simulink model "LQR"  (R2022b)
settings: Solver=VariableStepAuto  StartTime=0.0  StopTime=20  RelTol=1e-3
values from neighbouring files (symbols this model uses):
  B = [0 0 0 0;          1/Jx 0 0 0;          0 0 0 0 ... (first row only)    [config.m]
  g = 9.8    [config.m]
  Jx = 2*Mc*R^2/5 + 2*m*l^2    (= 0.0448)    [config.m]
  Jy = 2*Mc*R^2/5 + 2*m*l^2    (= 0.0448)    [config.m]
  Jz = 2*Mc*R^2/5 + 4*m*l^2    (= 0.0808)    [config.m]
  M = Mc + 4*m    (= 3)    [config.m]
undefined symbols (not defined in the file or in its folder): K_lqr
settings Model: Creator=cxk  LastModifiedBy=cxk

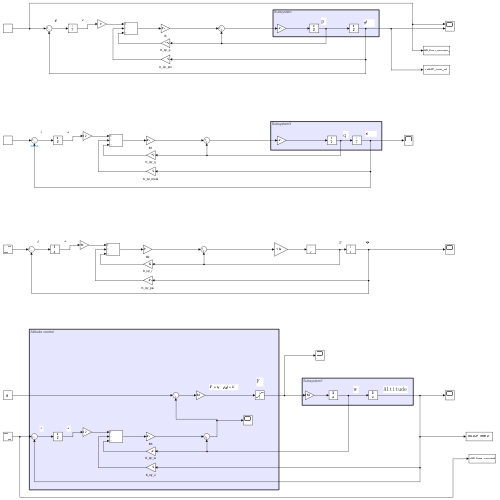
[thumbnail: Simulink's stored preview of the top-level diagram]
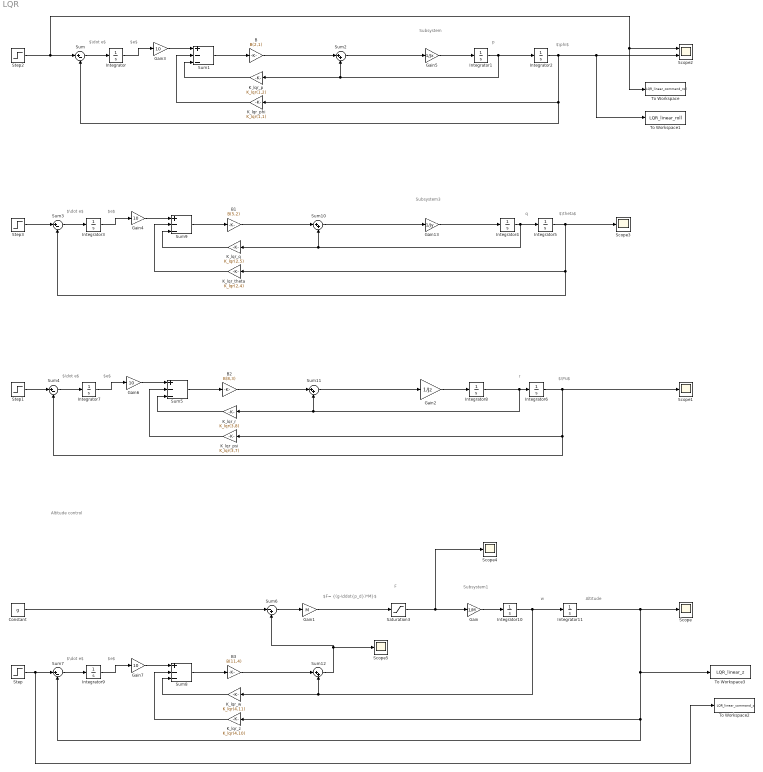
== system LQR ==
  note: Subsystem3
  note: Subsystem
  note: Altitude control
  note: Altitude
  note: $F= {(g-\ddot{p_d})*M}$
  note: Subsystem1
  note: w
  note: F
  note: $\Psi$
  note: r
  note: $\dot e$
  note: $e$
  note: p
  note: $\phi$
  note: $\theta$
  note: q
  note: $\dot e$
  note: $e$
  note: $\dot e$
  note: $e$
  note: $\dot e$
  note: $e$
  B : Gain  Gain=B(2,1)
  B1 : Gain  Gain=B(5,2)
  B2 : Gain  Gain=B(8,3)
  B3 : Gain  Gain=B(11,4)
  Constant : Constant  Value=g
  Gain : Gain  Gain=1/M
  Gain1 : Gain  Gain=M
  Gain13 : Gain  Gain=1/Jy
  Gain2 : Gain  Gain=1/Jz
  Gain{3..4,6..7} (4 alike) : Gain  Gain=10
  Gain5 : Gain  Gain=1/Jx
  Integrator{,1..11} (12 alike) : Integrator
  K_lqr_p : Gain  Gain=K_lqr(1,2)
  K_lqr_phi : Gain  Gain=K_lqr(1,1)
  K_lqr_psi : Gain  Gain=K_lqr(3,7)
  K_lqr_q : Gain  Gain=K_lqr(2,5)
  K_lqr_r : Gain  Gain=K_lqr(3,8)
  K_lqr_theta : Gain  Gain=K_lqr(2,4)
  K_lqr_w : Gain  Gain=K_lqr(4,11)
  K_lqr_z : Gain  Gain=K_lqr(4,10)
  Saturation3 : Saturate  UpperLimit=g*M*10  LowerLimit=-2.97*M*10
  Scope{,1,3..5} (5 alike) : Scope
  Scope2 : Scope  NumInputPorts=2
  Step : Step  After=-3  SampleTime=0
  Step1 : Step  SampleTime=0
  Step2 : Step  After=0.68  SampleTime=0
  Step3 : Step  After=0.68  SampleTime=0
  Sum{,3..4,7} (4 alike) : Sum  Inputs=|+-
  Sum{1,5,8..9} (4 alike) : Sum  Inputs=+--
  Sum{2,10..12} (4 alike) : Sum  Inputs=|++
  Sum6 : Sum  Inputs=|-+
  To Workspace : ToWorkspace  VariableName=LQR_linear_command_roll  SaveFormat=Timeseries  SampleTime=-1
  To Workspace1 : ToWorkspace  VariableName=LQR_linear_roll  SaveFormat=Timeseries  SampleTime=-1
  To Workspace2 : ToWorkspace  VariableName=LQR_linear_command_z  SaveFormat=Timeseries  SampleTime=-1
  To Workspace3 : ToWorkspace  VariableName=LQR_linear_z  SaveFormat=Timeseries  SampleTime=-1
  wires:
  Constant/1 -> Sum6/1
  Saturation3/1 -> Scope4/1, Gain/1
  Gain1/1 -> Saturation3/1
  Gain/1 -> Integrator10/1
  Sum6/1 -> Gain1/1
  Gain2/1 -> Integrator8/1
  Step2/1 -> To Workspace/1, Scope2/1, Sum/1
  Integrator2/1 -> K_lqr_phi/1, Sum/2, To Workspace1/1, Scope2/2
  Sum/1 -> Integrator/1
  Integrator/1 -> Gain3/1
  Gain3/1 -> Sum1/1
  K_lqr_phi/1 -> Sum1/2
  Sum1/1 -> B/1
  Integrator1/1 -> Sum2/2, K_lqr_p/1, Integrator2/1
  Sum2/1 -> Gain5/1
  B/1 -> Sum2/1
  K_lqr_p/1 -> Sum1/3
  Gain13/1 -> Integrator4/1
  Step3/1 -> Sum3/1
  Integrator4/1 -> Integrator5/1, Sum10/2, K_lqr_q/1
  K_lqr_q/1 -> Sum9/3
  Sum10/1 -> Gain13/1
  Sum3/1 -> Integrator3/1
  Integrator3/1 -> Gain4/1
  B1/1 -> Sum10/1
  Sum9/1 -> B1/1
  K_lqr_theta/1 -> Sum9/2
  Integrator5/1 -> K_lqr_theta/1, Sum3/2, Scope3/1
  Gain4/1 -> Sum9/1
  Gain5/1 -> Integrator1/1
  Step1/1 -> Sum4/1
  Integrator8/1 -> Sum11/2, K_lqr_r/1, Integrator6/1
  K_lqr_r/1 -> Sum5/3
  Sum11/1 -> Gain2/1
  Sum4/1 -> Integrator7/1
  Integrator7/1 -> Gain6/1
  B2/1 -> Sum11/1
  Sum5/1 -> B2/1
  K_lqr_psi/1 -> Sum5/2
  Integrator6/1 -> Sum4/2, K_lqr_psi/1, Scope1/1
  Gain6/1 -> Sum5/1
  Integrator10/1 -> Sum12/2, K_lqr_w/1, Integrator11/1
  K_lqr_w/1 -> Sum8/3
  Sum12/1 -> Sum6/2, Scope5/1
  Sum7/1 -> Integrator9/1
  Integrator9/1 -> Gain7/1
  B3/1 -> Sum12/1
  Sum8/1 -> B3/1
  K_lqr_z/1 -> Sum8/2
  Gain7/1 -> Sum8/1
  Integrator11/1 -> Sum7/2, K_lqr_z/1, To Workspace3/1, Scope/1
  Step/1 -> To Workspace2/1, Sum7/1
